simulink model "simulink1"  (R2020a)
settings: Solver=VariableStepAuto  StartTime=0.0  StopTime=10.0  RelTol=1e-3
settings Model: Creator=5111s  LastModifiedBy=5111s

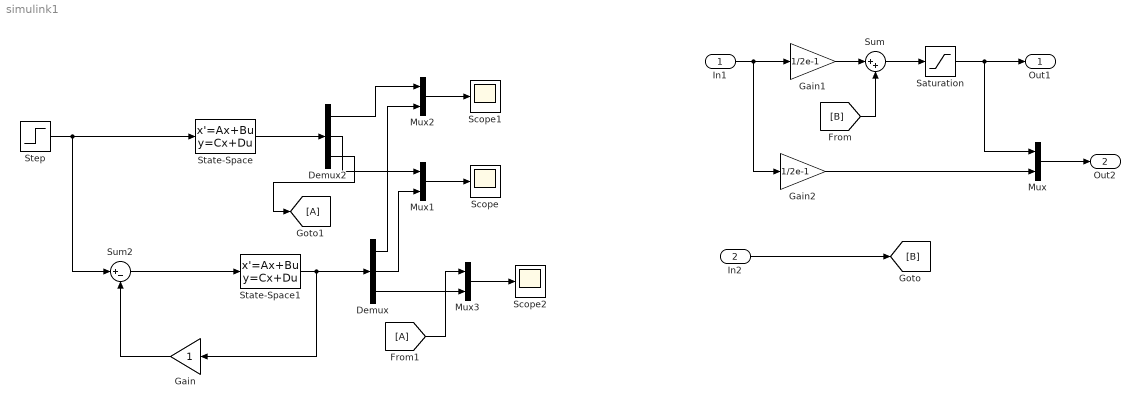
== system simulink1 ==
  In1 : Inport
  In2 : Inport  Port=2
  Demux : Demux  Outputs=3
  Demux2 : Demux  Outputs=3
  Gain : Gain
  Gain1 : Gain  Gain=1/2e-1
  Gain2 : Gain  Gain=1/2e-1
  Mux{,1..3} (4 alike) : Mux  Inputs=2
  Saturation : Saturate  UpperLimit=5
  Scope : Scope
  Scope1 : Scope
  Scope2 : Scope
  State-Space : StateSpace  InitialCondition=0
  State-Space1 : StateSpace  InitialCondition=0
  Step : Step  SampleTime=0
  Sum : Sum  Inputs=|++
  Sum2 : Sum  Inputs=|+-
  Out1 : Outport
  Out2 : Outport  Port=2
  wires:
  In1/1 -> Gain2/1, Gain1/1
  Saturation/1 -> Mux/1, Out1/1
  Gain2/1 -> Mux/2
  Mux/1 -> Out2/1
  [B] -> Sum/2
  Gain1/1 -> Sum/1
  Sum/1 -> Saturation/1
  In2/1 -> [B]
  Step/1 -> Sum2/1, State-Space/1
  Sum2/1 -> State-Space1/1
  State-Space1/1 -> Gain/1, Demux/1
  Gain/1 -> Sum2/2
  State-Space/1 -> Demux2/1
  Demux2/3 -> [A]
  Demux2/2 -> Mux1/1
  Demux/2 -> Mux1/2
  Demux2/1 -> Mux2/1
  Demux/1 -> Mux2/2
  Demux/3 -> Mux3/2
  [A] -> Mux3/1
  Mux1/1 -> Scope/1
  Mux2/1 -> Scope1/1
  Mux3/1 -> Scope2/1
